simulink model "HW7_v1"  (R2019b)
settings: Solver=VariableStepAuto  StartTime=0.0  StopTime=15  RelTol=1e-3
values from neighbouring files (symbols this model uses):
  A1 = [0 1;        0 0]    [HW7_v1.m]
  A1_wiener = [0 1 ;               0 0]    [HW7_v1.m]
  A2 = [0 1 0 0;        0 0 0 0;        0 0 0 1;       -9.81 0 0 0]    [HW7_v1.m]
  A2_cont = [0]    [HW7_v1.m]
  A3 = [0 1 0 0;        0 0 0 0;        0 0 0 1;       9.81 0 0 0]    [HW7_v1.m]
  A4 = [0 1;        0 0]    [HW7_v1.m]
  B1 = [0;      -0.067]    [HW7_v1.m]
  B1_wiener = [0;               1]    [HW7_v1.m]
  B2 = [0;        0.1442 ... (first row only)    [HW7_v1.m]
  B2_cont = [1]    [HW7_v1.m]
  B3 = [0;        0.1774;        0;        0]    [HW7_v1.m]
  B4 = [0;       0.1728]    [HW7_v1.m]
  C1 = [1 0]    [HW7_v1.m]
  C1_wiener = [1 0]    [HW7_v1.m]
  C2 = [1 0 0 0;        0 1 0 0;        0 0 1 0;        0 0 0 1]    [HW7_v1.m]
  C2_cont = [1]    [HW7_v1.m]
  C3 = [1 0 0 0;        0 1 0 0;        0 0 1 0;        0 0 0 1]    [HW7_v1.m]
  C4 = [1 0;        0 1]    [HW7_v1.m]
  D1 = [0]    [HW7_v1.m]
  D1_wiener = [0]    [HW7_v1.m]
  D2 = [0;        0;        0;        0]    [HW7_v1.m]
  D2_cont = [0]    [HW7_v1.m]
  D3 = [0;        0;        0;        0]    [HW7_v1.m]
  D4 = [0;       0]    [HW7_v1.m]
  Kx1 = K1(2:3)    [HW7_v1.m]
  L1 = lqe(A1_cont, G1, C1_cont, Q1, R1, N1)    [HW7_v1.m]
  L2 = lqe(A2_cont, G2, C2_cont, Q2, R2, N2)    [HW7_v1.m]
  L3 = lqe(A2_cont, G2, C2_cont, Q3, R3, N3)    [HW7_v1.m]
  L4 = lqe(A2_cont, G2, C2_cont, Q4, R4, N4)    [HW7_v1.m]
  L5 = lqe(A2_cont, G2, C2_cont, Q5, R5, N5)    [HW7_v1.m]
  M_inv = inv(M_motor)    [HW7_v1.m]
  M_motor = [1, 1, 1, -1;             1, 1, -1, 1;             1, -1, -1, -1;             1, -1, 1, 1 ]    [HW7_v1.m]
  tau2 = eval(max(solve(1/sqrt((tau2*2*pi*10)^2+1^2) == 1/sqrt(2), tau2)))    [HW7_v1.m]
  V = 5    [HW7_v1.m]
  V0 = 5    [HW7_v1.m]
undefined symbols (not defined in the file or in its folder): DiscIntNeverNeededParam, K2, K3, K4
settings Model: Creator=cwhipp  LastModifiedBy=cwhipp

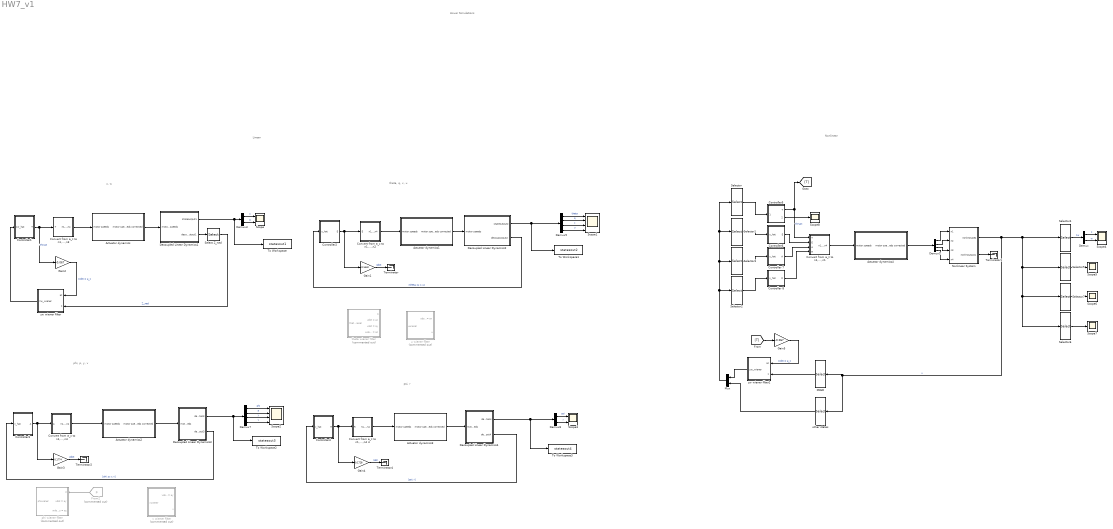
== system HW7_v1 ==
  note: Hover Simulations
  note: Nonlinear
  note: Linear
  note: z, w
  note: theta, q, x, u
  note: phi, p, y, v
  note: psi, r
  Actuator dynamics : Subsystem
  Actuator dynamics1 : Subsystem
  Actuator dynamics2 : Subsystem
  Actuator dynamics3 : Subsystem
  Actuator dynamics4 : Subsystem
  Controller 7 : Subsystem
  Controller 8 : Subsystem
  Controller1 : Subsystem
  Controller2 : Subsystem
  Controller3 : Subsystem
  Controller4 : Subsystem
  Controller5 : Subsystem
  Controller6 : Subsystem
  Convert from a_z to n1,...,n1 : Subsystem
  Convert from a_z to n1,...,n2 : Subsystem
  Convert from a_z to n1,...,n3 : Subsystem
  Convert from a_z to n1,...,n4 : Subsystem
  Convert from a_z to n1,...,n4 4 : Subsystem
  Decoupled Linear Dynamics1 : Subsystem
  Decoupled Linear Dynamics2 : Subsystem
  Decoupled Linear Dynamics3 : Subsystem
  "Decoupled Linear Dynamics4 " : Subsystem
  Demux : Demux  Outputs=2
  Demux1 : Demux
  Demux3 : Demux  Outputs=2
  Demux5 : Demux
  Demux7 : Demux
  Demux8 : Demux  Outputs=2
  From2 : From  Commented=on  GotoTag=p  TagVisibility=global
  Gain1 : Gain  Gain=0.1442
  Gain2 : Gain  Gain=-0.067
  Gain3 : Gain  Gain=0.1774
  Gain4 : Gain  Gain=0.1728
  Gain5 : Gain  Gain=-0.067
  Mux : Mux  Inputs=2
  Nonlinear System : Subsystem
  Scope : Scope  NumInputPorts=2
  Scope1 : Scope  NumInputPorts=4
  Scope2 : Scope  NumInputPorts=4
  Scope3 : Scope  NumInputPorts=2
  Scope4 : Scope  NumInputPorts=2
  Scope{5..8} (4 alike) : Scope
  Select Z_ned : Selector  InputPortWidth=4  IndexOptions=Index vector (dialog)  Indices=[1]  OutputSizes=1
  Selector : Selector  InputPortWidth=12  IndexOptions=Index vector (dialog)  Indices=[1 2]  OutputSizes=1
  Selector1 : Selector  InputPortWidth=12  IndexOptions=Index vector (dialog)  Indices=[3 4 5 6]  OutputSizes=1
  Selector2 : Selector  InputPortWidth=12  IndexOptions=Index vector (dialog)  Indices=[11 12]  OutputSizes=1
  Selector3 : Selector  InputPortWidth=12  IndexOptions=Index vector (dialog)  Indices=[7 8 9 10]  OutputSizes=1
  Selector4 : Selector  InputPortWidth=12  IndexOptions=Index vector (dialog)  Indices=[1 2]  OutputSizes=1
  Selector5 : Selector  InputPortWidth=12  IndexOptions=Index vector (dialog)  Indices=[3 4 5 6]  OutputSizes=1
  Selector6 : Selector  InputPortWidth=12  IndexOptions=Index vector (dialog)  Indices=[11 12]  OutputSizes=1
  Selector7 : Selector  InputPortWidth=12  IndexOptions=Index vector (dialog)  Indices=[7 8 9 10]  OutputSizes=1
  Terminator{,1..2,4} (4 alike) : Terminator
  To Workspace : ToWorkspace  VariableName=statesout1  SaveFormat=Timeseries  SampleTime=-1
  To Workspace1 : ToWorkspace  VariableName=statesout2  SaveFormat=Timeseries  SampleTime=-1
  To Workspace2 : ToWorkspace  VariableName=statesout3  SaveFormat=Timeseries  SampleTime=-1
  To Workspace3 : ToWorkspace  VariableName=statesout4  SaveFormat=Timeseries  SampleTime=-1
  ZNED : Selector  InputPortWidth=12  IndexOptions=Index vector (dialog)  Indices=[1]  OutputSizes=1
  other states : Selector  InputPortWidth=12  IndexOptions=Index vector (dialog)  Indices=[3 4 5 6 7 8 9 10 11 12]  OutputSizes=1
  phi wiener filter : Subsystem  Commented=on
  theta wiener filter : Subsystem  Commented=on
  u wiener filter : Subsystem  Commented=on
  v wiener filter : Subsystem  Commented=on
  zw wiener filter : Subsystem
  zw wiener filter2 : Subsystem
  wires:
  Gain5/1 -> zw wiener filter2/1(az)  "wdot = a_z"
  Demux1/1 -> Nonlinear System/1("n1 ")
  Demux1/2 -> Nonlinear System/2(n2)
  Demux1/3 -> Nonlinear System/3(n3)
  Demux1/4 -> Nonlinear System/4(n4)
  Controller1/1(T) -> Convert from a_z to n1,...,n3/1(T), Gain2/1  "thrust"
  Gain2/1 -> zw wiener filter/1(az)  "wdot = a_z"
  Select Z_ned/1 -> zw wiener filter/2(z)  "Z_ned"
  zw wiener filter/1(zw_wiener) -> Controller1/1(zw_hat)
  Decoupled Linear Dynamics1/2(decoupoutput1) -> Select Z_ned/1
  Decoupled Linear Dynamics2/2(decoupoutput2) -> Controller2/1(x_hat)  "[theta; q; x; u]"
  Controller2/1(E) -> Convert from a_z to n1,...,n2/1(E), Gain1/1
  Convert from a_z to n1,...,n2/1(n1,...,n4) -> Actuator dynamics1/1(motor speeds)
  Gain1/1 -> Terminator/1  "qdot"
  Decoupled Linear Dynamics3/2(decoupoutput3) -> Controller3/1(x_hat)  "[phi; p; y; v]"
  Gain3/1 -> Terminator2/1  "pdot"
  Convert from a_z to n1,...,n4/1(n1,...,n4) -> Actuator dynamics2/1(motor speeds)
  Controller3/1(A) -> Convert from a_z to n1,...,n4/1(A), Gain3/1
  From2/1 -> phi wiener filter/1(p)
  Controller4/1(R) -> Convert from a_z to n1,...,n4 4/1(R), Gain4/1
  Gain4/1 -> Terminator4/1  "rdot"
  Convert from a_z to n1,...,n4 4/1(n1,...,n4) -> Actuator dynamics3/1(motor speeds)
  "Decoupled Linear Dynamics4 "/2(decoupoutput4) -> Controller4/1(x_hat)  "[psi; r]"
  Decoupled Linear Dynamics1/1(stateoutput1) -> To Workspace/1, Demux3/1
  Demux3/1 -> Scope/1  "z"
  Demux3/2 -> Scope/2  "w"
  Demux5/4 -> Scope1/4  "u"
  Demux5/3 -> Scope1/3  "x"
  Demux5/2 -> Scope1/2  "q"
  Demux5/1 -> Scope1/1  "theta"
  Decoupled Linear Dynamics2/1(stateoutput2) -> To Workspace1/1, Demux5/1
  Demux7/2 -> Scope2/2  "p"
  Demux7/4 -> Scope2/4  "v"
  Demux7/1 -> Scope2/1  "phi"
  Demux7/3 -> Scope2/3  "y"
  Decoupled Linear Dynamics3/1(decoupstates3) -> To Workspace2/1, Demux7/1
  Demux8/2 -> Scope3/2  "r"
  Demux8/1 -> Scope3/1  "psi"
  "Decoupled Linear Dynamics4 "/1(decoupstates4) -> To Workspace3/1, Demux8/1
  Convert from a_z to n1,...,n3/1(n1,...,n4) -> Actuator dynamics/1(motor speeds)
  Actuator dynamics/1(motor speeds corrected) -> Decoupled Linear Dynamics1/1(motor speeds)
  Actuator dynamics1/1(motor speeds corrected) -> Decoupled Linear Dynamics2/1(motor speeds)
  Actuator dynamics2/1(motor speeds corrected) -> Decoupled Linear Dynamics3/1(motor speeds)
  Actuator dynamics3/1(motor speeds corrected) -> "Decoupled Linear Dynamics4 "/1(motor speeds)
  [T] -> Gain5/1
  Controller6/1(E) -> Convert from a_z to n1,...,n1/2(E)
  Controller 7/1(A) -> Convert from a_z to n1,...,n1/3(A)
  Controller 8/1(R) -> Convert from a_z to n1,...,n1/4(R)
  Selector1/1 -> Controller6/1(x_hat)
  Selector3/1 -> Controller 7/1(x_hat)
  Selector2/1 -> Controller 8/1(x_hat)
  Nonlinear System/2(nonlinoutputs) -> Terminator1/1
  ZNED/1 -> zw wiener filter2/2(z)
  zw wiener filter2/1(zw_wiener) -> Mux/1
  other states/1 -> Mux/2
  Mux/1 -> Selector/1, Selector1/1, Selector3/1, Selector2/1
  Nonlinear System/1("nonlinstates ") -> other states/1, ZNED/1, Selector6/1, Selector7/1, Selector5/1, Selector4/1  "x"
  Convert from a_z to n1,...,n1/1(n1,...,n4) -> Actuator dynamics4/1(motor speeds)
  Actuator dynamics4/1(motor speeds corrected) -> Demux1/1
  Selector4/1 -> Demux/1  "zw"
  Selector5/1 -> Scope5/1
  Selector7/1 -> Scope6/1
  Selector6/1 -> Scope7/1
  Controller5/1(T) -> Convert from a_z to n1,...,n1/1(T), [T]  "thrust"
  Selector/1 -> Controller5/1(zw_hat)
  Controller5/2(desired states) -> Scope8/1
  Demux/1 -> Scope4/1  "z"
  Demux/2 -> Scope4/2  "w"

== system HW7_v1/Actuator dynamics ==
  motor speeds : Inport
  30ms delay : TransportDelay  DelayTime=30e-3
  Demux : Demux
  Mux : Mux
  Saturation4 : Saturate  UpperLimit=500  LowerLimit=10
  Sum2 : Sum  Inputs=++|
  Transfer Fcn : TransferFcn  Denominator=[tau2 1]
  Transfer Fcn1 : TransferFcn  Denominator=[tau2 1]
  Transfer Fcn2 : TransferFcn  Denominator=[tau2 1]
  actuator transfer function : TransferFcn  Denominator=[tau2 1]
  speed correction : Constant  Value=299
  voltage correction : Gain  Gain=V/V0
  voltage error : Gain  Gain=V/V0
  motor speeds corrected : Outport
  wires:
  speed correction/1 -> Sum2/1
  voltage correction/1 -> voltage error/1
  Sum2/1 -> Saturation4/1
  Demux/2 -> Transfer Fcn1/1
  30ms delay/1 -> Demux/1
  Demux/4 -> actuator transfer function/1
  Demux/1 -> Transfer Fcn/1
  Demux/3 -> Transfer Fcn2/1
  voltage error/1 -> 30ms delay/1
  motor speeds/1 -> voltage correction/1
  Saturation4/1 -> motor speeds corrected/1
  Transfer Fcn/1 -> Mux/1
  Transfer Fcn1/1 -> Mux/2
  Transfer Fcn2/1 -> Mux/3
  actuator transfer function/1 -> Mux/4
  Mux/1 -> Sum2/2

== system HW7_v1/Actuator dynamics1 ==
  motor speeds : Inport
  30ms delay : TransportDelay  DelayTime=30e-3
  Demux : Demux
  Mux : Mux
  Saturation4 : Saturate  UpperLimit=500  LowerLimit=10
  Sum2 : Sum  Inputs=++|
  Transfer Fcn : TransferFcn  Denominator=[tau2 1]
  Transfer Fcn1 : TransferFcn  Denominator=[tau2 1]
  Transfer Fcn2 : TransferFcn  Denominator=[tau2 1]
  actuator transfer function : TransferFcn  Denominator=[tau2 1]
  speed correction : Constant  Value=299
  voltage correction : Gain  Gain=V/V0
  voltage error : Gain  Gain=V/V0
  motor speeds corrected : Outport
  wires:
  speed correction/1 -> Sum2/1
  voltage correction/1 -> voltage error/1
  Sum2/1 -> Saturation4/1
  Demux/2 -> Transfer Fcn1/1
  30ms delay/1 -> Demux/1
  Demux/4 -> actuator transfer function/1
  Demux/1 -> Transfer Fcn/1
  Demux/3 -> Transfer Fcn2/1
  voltage error/1 -> 30ms delay/1
  motor speeds/1 -> voltage correction/1
  Saturation4/1 -> motor speeds corrected/1
  Transfer Fcn/1 -> Mux/1
  Transfer Fcn1/1 -> Mux/2
  Transfer Fcn2/1 -> Mux/3
  actuator transfer function/1 -> Mux/4
  Mux/1 -> Sum2/2

== system HW7_v1/Actuator dynamics2 ==
  motor speeds : Inport
  30ms delay : TransportDelay  DelayTime=30e-3
  Demux : Demux
  Mux : Mux
  Saturation4 : Saturate  UpperLimit=500  LowerLimit=10
  Sum2 : Sum  Inputs=++|
  Transfer Fcn : TransferFcn  Denominator=[tau2 1]
  Transfer Fcn1 : TransferFcn  Denominator=[tau2 1]
  Transfer Fcn2 : TransferFcn  Denominator=[tau2 1]
  actuator transfer function : TransferFcn  Denominator=[tau2 1]
  speed correction : Constant  Value=299
  voltage correction : Gain  Gain=V/V0
  voltage error : Gain  Gain=V/V0
  motor speeds corrected : Outport
  wires:
  speed correction/1 -> Sum2/1
  voltage correction/1 -> voltage error/1
  Sum2/1 -> Saturation4/1
  Demux/2 -> Transfer Fcn1/1
  30ms delay/1 -> Demux/1
  Demux/4 -> actuator transfer function/1
  Demux/1 -> Transfer Fcn/1
  Demux/3 -> Transfer Fcn2/1
  voltage error/1 -> 30ms delay/1
  motor speeds/1 -> voltage correction/1
  Saturation4/1 -> motor speeds corrected/1
  Transfer Fcn/1 -> Mux/1
  Transfer Fcn1/1 -> Mux/2
  Transfer Fcn2/1 -> Mux/3
  actuator transfer function/1 -> Mux/4
  Mux/1 -> Sum2/2

== system HW7_v1/Actuator dynamics3 ==
  motor speeds : Inport
  30ms delay : TransportDelay  DelayTime=30e-3
  Demux : Demux
  Mux : Mux
  Saturation4 : Saturate  UpperLimit=500  LowerLimit=10
  Sum2 : Sum  Inputs=++|
  Transfer Fcn : TransferFcn  Denominator=[tau2 1]
  Transfer Fcn1 : TransferFcn  Denominator=[tau2 1]
  Transfer Fcn2 : TransferFcn  Denominator=[tau2 1]
  actuator transfer function : TransferFcn  Denominator=[tau2 1]
  speed correction : Constant  Value=299
  voltage correction : Gain  Gain=V/V0
  voltage error : Gain  Gain=V/V0
  motor speeds corrected : Outport
  wires:
  speed correction/1 -> Sum2/1
  voltage correction/1 -> voltage error/1
  Sum2/1 -> Saturation4/1
  Demux/2 -> Transfer Fcn1/1
  30ms delay/1 -> Demux/1
  Demux/4 -> actuator transfer function/1
  Demux/1 -> Transfer Fcn/1
  Demux/3 -> Transfer Fcn2/1
  voltage error/1 -> 30ms delay/1
  motor speeds/1 -> voltage correction/1
  Saturation4/1 -> motor speeds corrected/1
  Transfer Fcn/1 -> Mux/1
  Transfer Fcn1/1 -> Mux/2
  Transfer Fcn2/1 -> Mux/3
  actuator transfer function/1 -> Mux/4
  Mux/1 -> Sum2/2

== system HW7_v1/Actuator dynamics4 ==
  motor speeds : Inport
  30ms delay : TransportDelay  DelayTime=30e-3
  Demux : Demux
  Mux : Mux
  Saturation4 : Saturate  UpperLimit=500  LowerLimit=10
  Sum2 : Sum  Inputs=++|
  Transfer Fcn : TransferFcn  Denominator=[tau2 1]
  Transfer Fcn1 : TransferFcn  Denominator=[tau2 1]
  Transfer Fcn2 : TransferFcn  Denominator=[tau2 1]
  actuator transfer function : TransferFcn  Denominator=[tau2 1]
  speed correction : Constant  Value=299
  voltage correction : Gain  Gain=V/V0
  voltage error : Gain  Gain=V/V0
  motor speeds corrected : Outport
  wires:
  speed correction/1 -> Sum2/1
  voltage correction/1 -> voltage error/1
  Sum2/1 -> Saturation4/1
  Demux/2 -> Transfer Fcn1/1
  30ms delay/1 -> Demux/1
  Demux/4 -> actuator transfer function/1
  Demux/1 -> Transfer Fcn/1
  Demux/3 -> Transfer Fcn2/1
  voltage error/1 -> 30ms delay/1
  motor speeds/1 -> voltage correction/1
  Saturation4/1 -> motor speeds corrected/1
  Transfer Fcn/1 -> Mux/1
  Transfer Fcn1/1 -> Mux/2
  Transfer Fcn2/1 -> Mux/3
  actuator transfer function/1 -> Mux/4
  Mux/1 -> Sum2/2

== system HW7_v1/Controller 7 ==
  x_hat : Inport
  Sum : Sum  Inputs=+-|
  controller gain : Gain  Gain=K3  Multiplication=Matrix(K*u)
  desired velocity : Constant  Value=[0; 0; 0; 0]  SampleTime=0.05
  A : Outport
  wires:
  controller gain/1 -> A/1  "u = K(x-x)"
  x_hat/1 -> Sum/2
  Sum/1 -> controller gain/1
  desired velocity/1 -> Sum/1

== system HW7_v1/Controller 8 ==
  x_hat : Inport
  Sum : Sum  Inputs=+-|
  controller gain : Gain  Gain=K4  Multiplication=Matrix(K*u)
  desired velocity : Constant  Value=[0; 0]  SampleTime=0.05
  R : Outport
  wires:
  controller gain/1 -> R/1  "u = K(x-x)"
  x_hat/1 -> Sum/2
  Sum/1 -> controller gain/1
  desired velocity/1 -> Sum/1

== system HW7_v1/Controller1 ==
  zw_hat : Inport
  Constant1 : Constant  Value=1.5  SampleTime=0.05
  Gain : Gain  Gain=Kx1  Multiplication=Matrix(K*u)
  Gain1 : Gain  Gain=-1
  Mux : Mux  Inputs=2
  Scope : Scope
  Sum : Sum  Inputs=+-|
  Sum1 : Sum  Inputs=++|
  desired position : DiscretePulseGenerator  PulseType=Time based  Amplitude=-1.5  Period=10  PulseWidth=50
  desired velocity : Constant  Value=0  SampleTime=0.05
  T : Outport
  wires:
  Gain/1 -> T/1  "u = K(x-x)"
  zw_hat/1 -> Sum/2
  Sum/1 -> Gain/1
  Constant1/1 -> Sum1/1
  desired position/1 -> Sum1/2
  Sum1/1 -> Gain1/1
  Gain1/1 -> Mux/1
  desired velocity/1 -> Mux/2
  Mux/1 -> Scope/1, Sum/1

== system HW7_v1/Controller2 ==
  x_hat : Inport
  Sum : Sum  Inputs=+-|
  controller gain : Gain  Gain=K2  Multiplication=Matrix(K*u)
  desired velocity : Constant  Value=[0; 0; 0; 0]  SampleTime=0.05
  E : Outport
  wires:
  controller gain/1 -> E/1  "u = K(x-x)"
  x_hat/1 -> Sum/2
  Sum/1 -> controller gain/1
  desired velocity/1 -> Sum/1

== system HW7_v1/Controller3 ==
  x_hat : Inport
  Sum : Sum  Inputs=+-|
  controller gain : Gain  Gain=K3  Multiplication=Matrix(K*u)
  desired velocity : Constant  Value=[0; 0; 0; 0]  SampleTime=0.05
  A : Outport
  wires:
  controller gain/1 -> A/1  "u = K(x-x)"
  x_hat/1 -> Sum/2
  Sum/1 -> controller gain/1
  desired velocity/1 -> Sum/1

== system HW7_v1/Controller4 ==
  x_hat : Inport
  Sum : Sum  Inputs=+-|
  controller gain : Gain  Gain=K4  Multiplication=Matrix(K*u)
  desired velocity : Constant  Value=[0; 0]  SampleTime=0.05
  R : Outport
  wires:
  controller gain/1 -> R/1  "u = K(x-x)"
  x_hat/1 -> Sum/2
  Sum/1 -> controller gain/1
  desired velocity/1 -> Sum/1

== system HW7_v1/Controller5 ==
  zw_hat : Inport
  Constant1 : Constant  Value=1.5  SampleTime=0.05
  Gain : Gain  Gain=Kx1  Multiplication=Matrix(K*u)
  Gain1 : Gain  Gain=-1
  Mux : Mux  Inputs=2
  Sum : Sum  Inputs=+-|
  Sum1 : Sum  Inputs=++|
  desired position : DiscretePulseGenerator  PulseType=Time based  Amplitude=-1.5  Period=10  PulseWidth=50
  desired velocity : Constant  Value=0  SampleTime=0.05
  T : Outport
  desired states : Outport  Port=2
  wires:
  Gain/1 -> T/1  "u = K(x-x)"
  zw_hat/1 -> Sum/2
  Sum/1 -> Gain/1
  Constant1/1 -> Sum1/1
  desired position/1 -> Sum1/2
  Sum1/1 -> Gain1/1
  Gain1/1 -> Mux/1
  desired velocity/1 -> Mux/2
  Mux/1 -> Sum/1, desired states/1

== system HW7_v1/Controller6 ==
  x_hat : Inport
  Sum : Sum  Inputs=+-|
  controller gain : Gain  Gain=K2  Multiplication=Matrix(K*u)
  desired velocity : Constant  Value=[0; 0; 0; 0]  SampleTime=0.05
  E : Outport
  wires:
  controller gain/1 -> E/1  "u = K(x-x)"
  x_hat/1 -> Sum/2
  Sum/1 -> controller gain/1
  desired velocity/1 -> Sum/1

== system HW7_v1/Convert from a_z to n1,...,n1 ==
  T : Inport
  E : Inport  Port=2
  A : Inport  Port=3
  R : Inport  Port=4
  Convert fom TEAR to n1,..,n4 : Gain  Gain=M_motor  Multiplication=Matrix(K*u)
  Mux : Mux
  n1,...,n4 : Outport
  wires:
  Convert fom TEAR to n1,..,n4/1 -> n1,...,n4/1
  Mux/1 -> Convert fom TEAR to n1,..,n4/1
  T/1 -> Mux/1
  E/1 -> Mux/2
  A/1 -> Mux/3
  R/1 -> Mux/4

== system HW7_v1/Convert from a_z to n1,...,n2 ==
  E : Inport
  Constant : Constant  Value=0
  Convert fom TEAR to n1,..,n4 : Gain  Gain=M_motor  Multiplication=Matrix(K*u)
  Mux : Mux
  n1,...,n4 : Outport
  wires:
  Constant/1 -> Mux/4, Mux/1, Mux/3
  Convert fom TEAR to n1,..,n4/1 -> n1,...,n4/1
  Mux/1 -> Convert fom TEAR to n1,..,n4/1
  E/1 -> Mux/2

== system HW7_v1/Convert from a_z to n1,...,n3 ==
  T : Inport
  Constant : Constant  Value=0
  Convert fom TEAR to n1,..,n4 : Gain  Gain=M_motor  Multiplication=Matrix(K*u)
  Mux : Mux
  n1,...,n4 : Outport
  wires:
  Constant/1 -> Mux/4, Mux/3, Mux/2
  Convert fom TEAR to n1,..,n4/1 -> n1,...,n4/1
  Mux/1 -> Convert fom TEAR to n1,..,n4/1
  T/1 -> Mux/1

== system HW7_v1/Convert from a_z to n1,...,n4 ==
  A : Inport
  Constant : Constant  Value=0
  Convert fom TEAR to n1,..,n4 : Gain  Gain=M_motor  Multiplication=Matrix(K*u)
  Mux : Mux
  n1,...,n4 : Outport
  wires:
  Constant/1 -> Mux/4, Mux/2, Mux/1
  Convert fom TEAR to n1,..,n4/1 -> n1,...,n4/1
  Mux/1 -> Convert fom TEAR to n1,..,n4/1
  A/1 -> Mux/3

== system HW7_v1/Convert from a_z to n1,...,n4 4 ==
  R : Inport
  Constant : Constant  Value=0
  Convert fom TEAR to n1,..,n4 : Gain  Gain=M_motor  Multiplication=Matrix(K*u)
  Mux : Mux
  n1,...,n4 : Outport
  wires:
  Constant/1 -> Mux/3, Mux/2, Mux/1
  Convert fom TEAR to n1,..,n4/1 -> n1,...,n4/1
  Mux/1 -> Convert fom TEAR to n1,..,n4/1
  R/1 -> Mux/4

== system HW7_v1/Decoupled Linear Dynamics1 ==
  motor speeds : Inport
  B*u : Gain  Gain=B1  Multiplication=Matrix(K*u)
  Demux : Demux
  Gain : Gain  Gain=M_inv  Multiplication=Matrix(K*u)
  Gain2 : Gain  Gain=C1  Multiplication=Matrix(K*u)
  Gain3 : Gain  Gain=D1  Multiplication=Matrix(K*u)
  Gain69 : Gain  Gain=A1  Multiplication=Matrix(K*u)
  Integrator : Integrator
  Selector : Selector  InputPortWidth=4  IndexOptions=Index vector (dialog)  Indices=1  OutputSizes=1
  Sum : Sum  Inputs=|++
  Sum1 : Sum  Inputs=|++
  Sum4 : Sum  Inputs=-+|
  asdf : Scope  NumInputPorts=4
  change back to trim = 0 : Constant  Value=299
  stateoutput1 : Outport
  decoupoutput1 : Outport  Port=2
  wires:
  Sum/1 -> Integrator/1
  Gain69/1 -> Sum/2  "Ax"
  Gain3/1 -> Sum1/1  "Du"
  Sum1/1 -> decoupoutput1/1  "y"
  B*u/1 -> Sum/1
  Gain2/1 -> Sum1/2  "Cx"
  Selector/1 -> Gain3/1, B*u/1  "u"
  Gain/1 -> Selector/1
  Integrator/1 -> Gain2/1, stateoutput1/1, Gain69/1  "x"
  change back to trim = 0/1 -> Sum4/1
  Demux/1 -> asdf/1
  Demux/2 -> asdf/2
  Demux/3 -> asdf/3
  Sum4/1 -> Demux/1, Gain/1
  motor speeds/1 -> Sum4/2
  Demux/4 -> asdf/4

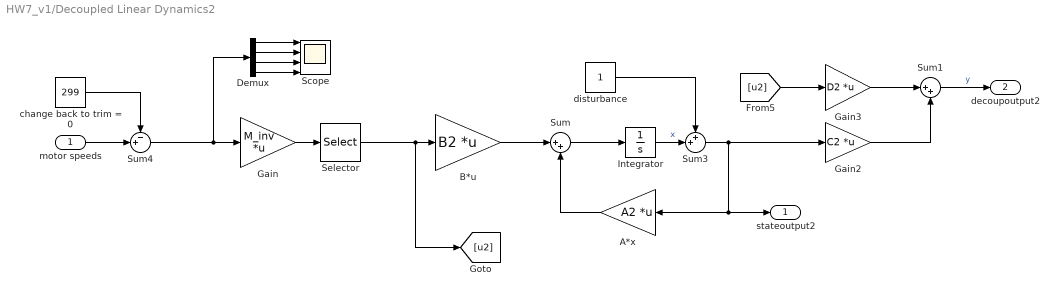
== system HW7_v1/Decoupled Linear Dynamics2 ==
  motor speeds : Inport
  A*x : Gain  Gain=A2  Multiplication=Matrix(K*u)
  B*u : Gain  Gain=B2  Multiplication=Matrix(K*u)
  Demux : Demux
  Gain : Gain  Gain=M_inv  Multiplication=Matrix(K*u)
  Gain2 : Gain  Gain=C2  Multiplication=Matrix(K*u)
  Gain3 : Gain  Gain=D2  Multiplication=Matrix(K*u)
  Integrator : Integrator
  Scope : Scope  NumInputPorts=4
  Selector : Selector  InputPortWidth=4  IndexOptions=Index vector (dialog)  Indices=2  OutputSizes=1
  Sum : Sum  Inputs=|++
  Sum1 : Sum  Inputs=|++
  Sum3 : Sum  Inputs=++|
  Sum4 : Sum  Inputs=-+|
  change back to trim = 0 : Constant  Value=299
  disturbance : Constant
  stateoutput2 : Outport
  decoupoutput2 : Outport  Port=2
  wires:
  Sum/1 -> Integrator/1
  A*x/1 -> Sum/2
  Gain3/1 -> Sum1/1
  Sum1/1 -> decoupoutput2/1  "y"
  B*u/1 -> Sum/1
  Gain2/1 -> Sum1/2
  [u2] -> Gain3/1
  Sum4/1 -> Demux/1, Gain/1
  Gain/1 -> Selector/1
  Selector/1 -> [u2], B*u/1
  change back to trim = 0/1 -> Sum4/1
  Demux/1 -> Scope/1
  Demux/2 -> Scope/2
  Demux/3 -> Scope/3
  Demux/4 -> Scope/4
  motor speeds/1 -> Sum4/2
  disturbance/1 -> Sum3/1
  Integrator/1 -> Sum3/2  "x"
  Sum3/1 -> stateoutput2/1, A*x/1, Gain2/1

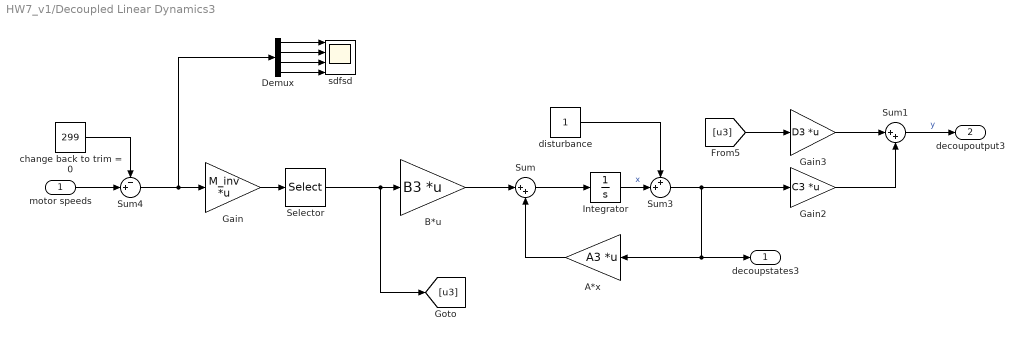
== system HW7_v1/Decoupled Linear Dynamics3 ==
  motor speeds : Inport
  A*x : Gain  Gain=A3  Multiplication=Matrix(K*u)
  B*u : Gain  Gain=B3  Multiplication=Matrix(K*u)
  Demux : Demux
  Gain : Gain  Gain=M_inv  Multiplication=Matrix(K*u)
  Gain2 : Gain  Gain=C3  Multiplication=Matrix(K*u)
  Gain3 : Gain  Gain=D3  Multiplication=Matrix(K*u)
  Integrator : Integrator
  Selector : Selector  InputPortWidth=4  IndexOptions=Index vector (dialog)  Indices=3  OutputSizes=1
  Sum : Sum  Inputs=|++
  Sum1 : Sum  Inputs=|++
  Sum3 : Sum  Inputs=++|
  Sum4 : Sum  Inputs=-+|
  change back to trim = 0 : Constant  Value=299
  disturbance : Constant
  sdfsd : Scope  NumInputPorts=4
  decoupstates3 : Outport
  decoupoutput3 : Outport  Port=2
  wires:
  Sum/1 -> Integrator/1
  A*x/1 -> Sum/2
  Gain3/1 -> Sum1/1
  Sum1/1 -> decoupoutput3/1  "y"
  B*u/1 -> Sum/1
  Gain2/1 -> Sum1/2
  [u3] -> Gain3/1
  Sum4/1 -> Demux/1, Gain/1
  Gain/1 -> Selector/1
  Selector/1 -> [u3], B*u/1
  change back to trim = 0/1 -> Sum4/1
  Demux/1 -> sdfsd/1
  Demux/2 -> sdfsd/2
  Demux/3 -> sdfsd/3
  Demux/4 -> sdfsd/4
  motor speeds/1 -> Sum4/2
  disturbance/1 -> Sum3/1
  Integrator/1 -> Sum3/2  "x"
  Sum3/1 -> decoupstates3/1, A*x/1, Gain2/1

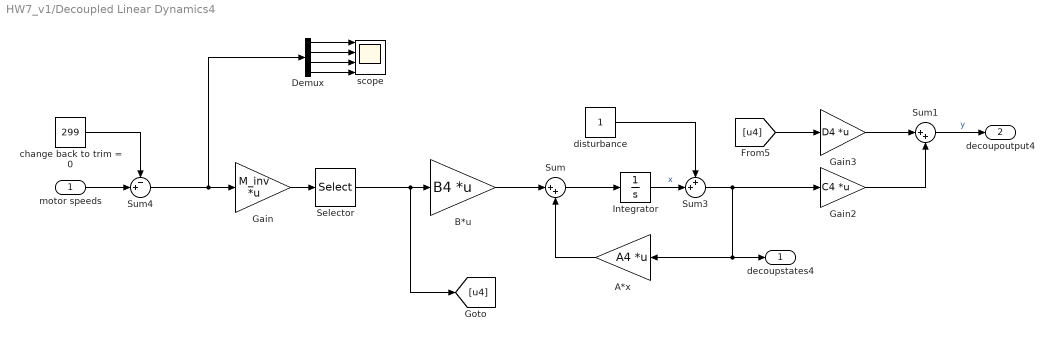
== system HW7_v1/Decoupled Linear Dynamics4  ==
  motor speeds : Inport
  A*x : Gain  Gain=A4  Multiplication=Matrix(K*u)
  B*u : Gain  Gain=B4  Multiplication=Matrix(K*u)
  Demux : Demux
  Gain : Gain  Gain=M_inv  Multiplication=Matrix(K*u)
  Gain2 : Gain  Gain=C4  Multiplication=Matrix(K*u)
  Gain3 : Gain  Gain=D4  Multiplication=Matrix(K*u)
  Integrator : Integrator
  Selector : Selector  InputPortWidth=4  IndexOptions=Index vector (dialog)  Indices=4  OutputSizes=1
  Sum : Sum  Inputs=|++
  Sum1 : Sum  Inputs=|++
  Sum3 : Sum  Inputs=++|
  Sum4 : Sum  Inputs=-+|
  change back to trim = 0 : Constant  Value=299
  disturbance : Constant
  scope : Scope  NumInputPorts=4
  decoupstates4 : Outport
  decoupoutput4 : Outport  Port=2
  wires:
  Sum/1 -> Integrator/1
  A*x/1 -> Sum/2
  Gain3/1 -> Sum1/1
  Sum1/1 -> decoupoutput4/1  "y"
  B*u/1 -> Sum/1
  Gain2/1 -> Sum1/2
  [u4] -> Gain3/1
  Sum4/1 -> Demux/1, Gain/1
  Gain/1 -> Selector/1
  Selector/1 -> [u4], B*u/1
  change back to trim = 0/1 -> Sum4/1
  Demux/1 -> scope/1
  Demux/2 -> scope/2
  Demux/3 -> scope/3
  Demux/4 -> scope/4
  Sum3/1 -> decoupstates4/1, A*x/1, Gain2/1
  motor speeds/1 -> Sum4/2
  disturbance/1 -> Sum3/1
  Integrator/1 -> Sum3/2  "x"

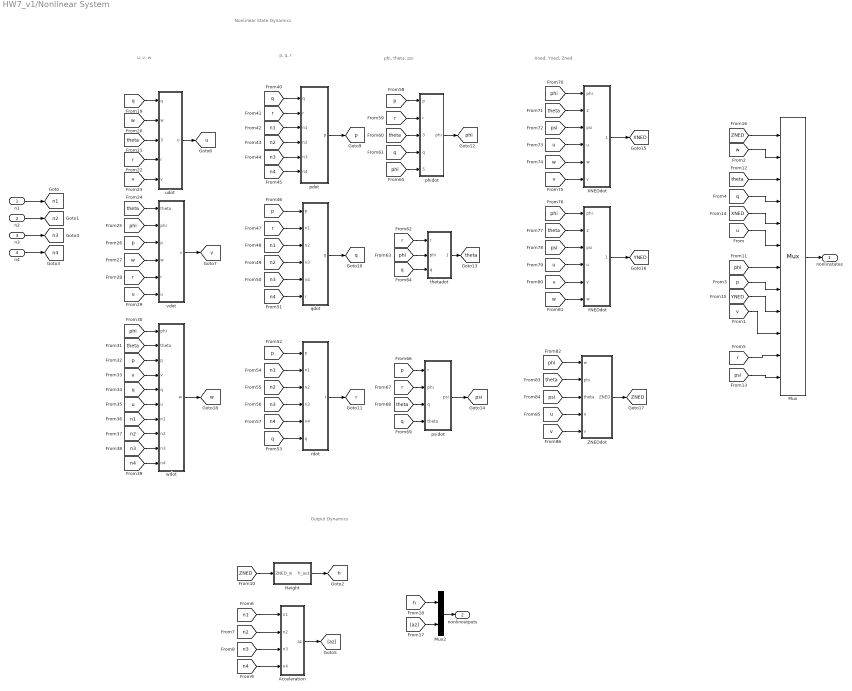
== system HW7_v1/Nonlinear System ==
  note: Output Dynamics
  note: Nonlinear State Dynamics
  note: p, q, r
  note: u, v, w
  note: phi, theta, psi
  note: Xned, Yned, Zned
  "n1 " : Inport
  n2 : Inport  Port=2
  n3 : Inport  Port=3
  n4 : Inport  Port=4
  Acceleration : Subsystem
  Height : Subsystem
  Mux : Mux  Inputs=12
  Mux2 : Mux  Inputs=2
  "XNEDdot " : Subsystem
  "YNEDdot " : Subsystem
  ZNEDdot : Subsystem
  pdot : Subsystem
  phidot : Subsystem
  "psidot " : Subsystem
  qdot : Subsystem
  rdot : Subsystem
  "thetadot " : Subsystem
  udot : Subsystem
  vdot : Subsystem
  "wdot " : Subsystem
  "nonlinstates " : Outport
  nonlinoutputs : Outport  Port=2
  tag scope: XNED=global, YNED=global, ZNED=global, h=global, n1=global, n2=global, n3=global, n4=global, p=global, phi=global, psi=global, q=global, r=global, theta=global, u=global, v=global, w=global
  wires:
  [n2] -> Acceleration/2(n2)
  [n1] -> Acceleration/1(n1)
  [n3] -> Acceleration/3(n3)
  Acceleration/1(az) -> [az]
  [n4] -> Acceleration/4(n4)
  [ZNED] -> Height/1("ZNED_in ")
  Height/1("h_out ") -> [h]
  Mux/1 -> "nonlinstates "/1
  [h] -> Mux2/1
  [az] -> Mux2/2
  Mux2/1 -> nonlinoutputs/1
  udot/1("u ") -> [u]
  [q] -> udot/1("q ")
  [w] -> udot/2("w ")
  [theta] -> udot/3(theta)
  [r] -> udot/4("r ")
  [v] -> udot/5(v)
  "n1 "/1 -> [n1]
  n2/1 -> [n2]
  n3/1 -> [n3]
  n4/1 -> [n4]
  [theta] -> vdot/1(theta)
  [phi] -> vdot/2(phi)
  [p] -> vdot/3(p)
  [w] -> vdot/4(w)
  [r] -> vdot/5(r)
  [u] -> vdot/6(u)
  vdot/1(v) -> [v]
  [phi] -> "wdot "/1(phi)
  [theta] -> "wdot "/2(theta)
  [p] -> "wdot "/3(p)
  [v] -> "wdot "/4(v)
  [q] -> "wdot "/5(q)
  [u] -> "wdot "/6(u)
  [n1] -> "wdot "/7(n1)
  [n2] -> "wdot "/8(n2)
  [n3] -> "wdot "/9(n3)
  [n4] -> "wdot "/10(n4)
  "wdot "/1(w) -> [w]
  [n1] -> pdot/3(n1)
  [r] -> pdot/2(r)
  [n2] -> pdot/4(n2)
  [q] -> pdot/1(q)
  [n3] -> pdot/5(n3)
  [n4] -> pdot/6(n4)
  [p] -> qdot/1(p)
  [r] -> qdot/2(n1)
  [n1] -> qdot/3(n2)
  [n2] -> qdot/4(n3)
  [n3] -> qdot/5(n4)
  [n4] -> qdot/6(r)
  qdot/1(q) -> [q]
  [p] -> rdot/1(p)
  [n1] -> rdot/2(n1)
  [n2] -> rdot/3(n2)
  [n3] -> rdot/4(n3)
  [n4] -> rdot/5(n4)
  [q] -> rdot/6(q)
  rdot/1(r) -> [r]
  [p] -> phidot/1(p)
  [r] -> phidot/2(r)
  [theta] -> phidot/3(theta)
  [q] -> phidot/4(q)
  phidot/1(phi) -> [phi]
  [q] -> "thetadot "/3(q)
  [r] -> "thetadot "/1(r)
  [phi] -> "thetadot "/2(phi)
  "thetadot "/1(theta) -> [theta]
  pdot/1(p) -> [p]
  [phi] -> phidot/5(phi in)
  [r] -> "psidot "/2(phi)
  [p] -> "psidot "/1(r)
  [theta] -> "psidot "/3(q)
  [q] -> "psidot "/4(theta)
  "psidot "/1(psi) -> [psi]
  [phi] -> "XNEDdot "/1(phi)
  [u] -> "XNEDdot "/4(u)
  [w] -> "XNEDdot "/5(w)
  [v] -> "XNEDdot "/6(v)
  [theta] -> "XNEDdot "/2(theta)
  [psi] -> "XNEDdot "/3(psi)
  "XNEDdot "/1(XNED) -> [XNED]
  [w] -> "YNEDdot "/6(w)
  [v] -> "YNEDdot "/5(v)
  [u] -> "YNEDdot "/4(u)
  [psi] -> "YNEDdot "/3(psi)
  [theta] -> "YNEDdot "/2(theta)
  "YNEDdot "/1(YNED) -> [YNED]
  [phi] -> "YNEDdot "/1(phi)
  [phi] -> ZNEDdot/1(w)
  [theta] -> ZNEDdot/2(phi)
  [psi] -> ZNEDdot/3(theta)
  [u] -> ZNEDdot/4(u)
  [v] -> ZNEDdot/5(v)
  ZNEDdot/1(ZNED) -> [ZNED]
  [r] -> Mux/11
  [psi] -> Mux/12
  [phi] -> Mux/7
  [p] -> Mux/8
  [YNED] -> Mux/9
  [v] -> Mux/10
  [u] -> Mux/6
  [XNED] -> Mux/5
  [q] -> Mux/4
  [theta] -> Mux/3
  [w] -> Mux/2
  [ZNED] -> Mux/1

== system HW7_v1/phi wiener filter ==
  p : Inport
  vdot = ay : Inport  Port=2
  wdotnobias = az : Inport  Port=3
  Discrete-Time Integrator3 : DiscreteIntegrator  IntegratorMethod=Integration: Backward Euler  SampleTime=-1  ICPrevOutput=DiscIntNeverNeededParam  ICPrevScaledInput=DiscIntNeverNeededParam
  Divide2 : Product  Inputs=*/
  Gain16 : Gain  Gain=D2_cont  Multiplication=Matrix(K*u)
  Gain17 : Gain  Gain=A2_cont  Multiplication=Matrix(K*u)
  Gain18 : Gain  Gain=B2_cont  Multiplication=Matrix(K*u)
  Gain19 : Gain  Gain=L4  Multiplication=Matrix(K*u)
  Gain20 : Gain  Gain=C2_cont  Multiplication=Matrix(K*u)
  Memory4 : Memory
  Sum15 : Sum  Inputs=|+-
  Sum16 : Sum  Inputs=|++
  Sum17 : Sum  Inputs=|++
  Sum18 : Sum  Inputs=|+-
  phiwiener : Outport
  wires:
  Gain18/1 -> Sum16/2  "Bu"
  Gain17/1 -> Sum16/1  "Axe"
  Gain19/1 -> Sum17/2  "L(y-Cx-Du)"
  Sum18/1 -> Gain19/1
  Discrete-Time Integrator3/1 -> Gain17/1, phiwiener/1, Gain20/1  "xe"
  wdotnobias = az/1 -> Divide2/2
  Memory4/1 -> Discrete-Time Integrator3/1
  vdot = ay/1 -> Divide2/1
  Divide2/1 -> Sum15/1  "phi"
  p/1 -> Gain16/1, Gain18/1  "u"
  Sum15/1 -> Sum18/1
  Sum16/1 -> Sum17/1
  Sum17/1 -> Memory4/1
  Gain16/1 -> Sum15/2  "Du"
  Gain20/1 -> Sum18/2  "Cx"

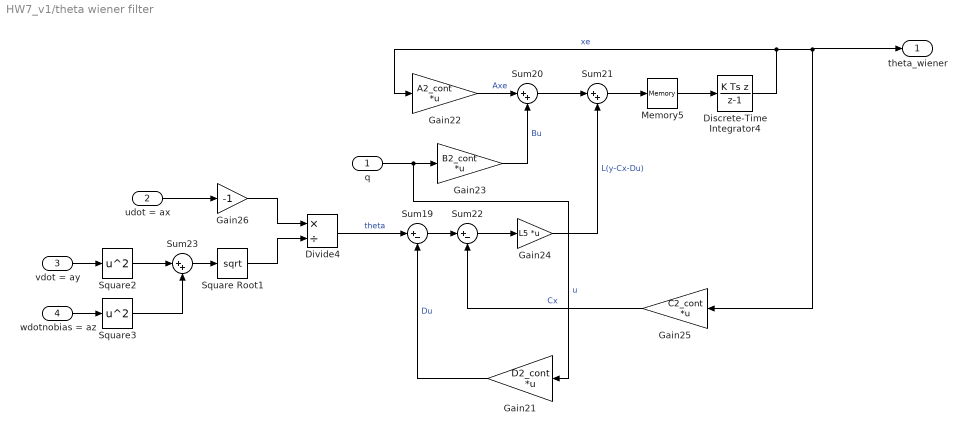
== system HW7_v1/theta wiener filter ==
  q : Inport
  udot = ax : Inport  Port=2
  vdot = ay : Inport  Port=3
  "wdotnobias = az " : Inport  Port=4
  Discrete-Time Integrator4 : DiscreteIntegrator  IntegratorMethod=Integration: Backward Euler  SampleTime=-1  ICPrevOutput=DiscIntNeverNeededParam  ICPrevScaledInput=DiscIntNeverNeededParam
  Divide4 : Product  Inputs=*/
  Gain21 : Gain  Gain=D2_cont  Multiplication=Matrix(K*u)
  Gain22 : Gain  Gain=A2_cont  Multiplication=Matrix(K*u)
  Gain23 : Gain  Gain=B2_cont  Multiplication=Matrix(K*u)
  Gain24 : Gain  Gain=L5  Multiplication=Matrix(K*u)
  Gain25 : Gain  Gain=C2_cont  Multiplication=Matrix(K*u)
  Gain26 : Gain  Gain=-1
  Memory5 : Memory
  Square Root1 : Sqrt  SaturateOnIntegerOverflow=on
  Square2 : Math  Operator=square  SignedPower=off  SaturateOnIntegerOverflow=on
  Square3 : Math  Operator=square  SignedPower=off  SaturateOnIntegerOverflow=on
  Sum19 : Sum  Inputs=|+-
  Sum20 : Sum  Inputs=|++
  Sum21 : Sum  Inputs=|++
  Sum22 : Sum  Inputs=|+-
  Sum23 : Sum  Inputs=|++
  theta_wiener : Outport
  wires:
  Sum23/1 -> Square Root1/1
  Sum22/1 -> Gain24/1
  q/1 -> Gain21/1, Gain23/1  "u"
  Square3/1 -> Sum23/2
  Discrete-Time Integrator4/1 -> Gain22/1, Gain25/1, theta_wiener/1  "xe"
  Gain24/1 -> Sum21/2  "L(y-Cx-Du)"
  Square2/1 -> Sum23/1
  Square Root1/1 -> Divide4/2
  Divide4/1 -> Sum19/1  "theta"
  "wdotnobias = az "/1 -> Square3/1
  vdot = ay/1 -> Square2/1
  Memory5/1 -> Discrete-Time Integrator4/1
  udot = ax/1 -> Gain26/1
  Sum20/1 -> Sum21/1
  Gain25/1 -> Sum22/2  "Cx"
  Sum21/1 -> Memory5/1
  Gain26/1 -> Divide4/1
  Gain21/1 -> Sum19/2  "Du"
  Gain22/1 -> Sum20/1  "Axe"
  Sum19/1 -> Sum22/1
  Gain23/1 -> Sum20/2  "Bu"

== system HW7_v1/u wiener filter ==
  udot = ax : Inport
  u : Inport  Port=2
  Discrete-Time Integrator1 : DiscreteIntegrator  IntegratorMethod=Integration: Backward Euler  SampleTime=-1  ICPrevOutput=DiscIntNeverNeededParam  ICPrevScaledInput=DiscIntNeverNeededParam
  Gain10 : Gain  Gain=D2_cont  Multiplication=Matrix(K*u)
  Gain5 : Gain  Gain=A2_cont  Multiplication=Matrix(K*u)
  Gain7 : Gain  Gain=B2_cont  Multiplication=Matrix(K*u)
  Gain8 : Gain  Gain=L2  Multiplication=Matrix(K*u)
  Gain9 : Gain  Gain=C2_cont  Multiplication=Matrix(K*u)
  Memory2 : Memory
  Sum10 : Sum  Inputs=|+-
  Sum6 : Sum  Inputs=|++
  Sum8 : Sum  Inputs=|++
  Sum9 : Sum  Inputs=|+-
  "uwiener " : Outport
  wires:
  Gain7/1 -> Sum6/2  "Bu"
  Discrete-Time Integrator1/1 -> Gain5/1, Gain9/1, "uwiener "/1  "xe"
  Memory2/1 -> Discrete-Time Integrator1/1
  u/1 -> Sum10/1
  Gain9/1 -> Sum9/2  "Cx"
  Sum6/1 -> Sum8/1
  Sum8/1 -> Memory2/1
  Gain8/1 -> Sum8/2  "L(y-Cx-Du)"
  Sum10/1 -> Sum9/1
  Sum9/1 -> Gain8/1
  udot = ax/1 -> Gain10/1, Gain7/1  "u"
  Gain5/1 -> Sum6/1  "Axe"
  Gain10/1 -> Sum10/2  "Du"

== system HW7_v1/v wiener filter ==
  vdot = ay : Inport
  v : Inport  Port=2
  Discrete-Time Integrator2 : DiscreteIntegrator  IntegratorMethod=Integration: Backward Euler  SampleTime=-1  ICPrevOutput=DiscIntNeverNeededParam  ICPrevScaledInput=DiscIntNeverNeededParam
  Gain11 : Gain  Gain=D2_cont  Multiplication=Matrix(K*u)
  Gain12 : Gain  Gain=A2_cont  Multiplication=Matrix(K*u)
  Gain13 : Gain  Gain=B2_cont  Multiplication=Matrix(K*u)
  Gain14 : Gain  Gain=L3  Multiplication=Matrix(K*u)
  Gain15 : Gain  Gain=C2_cont  Multiplication=Matrix(K*u)
  Memory3 : Memory
  Sum11 : Sum  Inputs=|+-
  Sum12 : Sum  Inputs=|++
  Sum13 : Sum  Inputs=|++
  Sum14 : Sum  Inputs=|+-
  vwiener : Outport
  wires:
  v/1 -> Sum11/1
  vdot = ay/1 -> Gain11/1, Gain13/1  "u"
  Sum14/1 -> Gain14/1
  Gain11/1 -> Sum11/2  "Du"
  Gain14/1 -> Sum13/2  "L(y-Cx-Du)"
  Discrete-Time Integrator2/1 -> Gain12/1, Gain15/1, vwiener/1  "xe"
  Sum11/1 -> Sum14/1
  Memory3/1 -> Discrete-Time Integrator2/1
  Sum13/1 -> Memory3/1
  Gain13/1 -> Sum12/2  "Bu"
  Gain12/1 -> Sum12/1  "Axe"
  Sum12/1 -> Sum13/1
  Gain15/1 -> Sum14/2  "Cx"

== system HW7_v1/zw wiener filter ==
  note: zw Wiener Filter
  az : Inport
  z : Inport  Port=2
  Discrete-Time Integrator : DiscreteIntegrator  SampleTime=-1  ICPrevOutput=DiscIntNeverNeededParam  ICPrevScaledInput=DiscIntNeverNeededParam
  Gain1 : Gain  Gain=A1_wiener  Multiplication=Matrix(K*u)
  Gain2 : Gain  Gain=B1_wiener  Multiplication=Matrix(K*u)
  Gain3 : Gain  Gain=L1  Multiplication=Matrix(K*u)
  Gain4 : Gain  Gain=C1_wiener  Multiplication=Matrix(K*u)
  Gain6 : Gain  Gain=D1_wiener  Multiplication=Matrix(K*u)
  Sum3 : Sum  Inputs=+++
  Sum7 : Sum  Inputs=-+-
  zw_wiener : Outport
  wires:
  Gain3/1 -> Sum3/3  "L(y-Cx-Du)"
  Gain1/1 -> Sum3/1  "Axe"
  Gain2/1 -> Sum3/2  "Bu"
  Discrete-Time Integrator/1 -> zw_wiener/1, Gain1/1, Gain4/1  "xe"
  Gain6/1 -> Sum7/1  "Du"
  az/1 -> Gain6/1, Gain2/1  "u = az"
  Sum7/1 -> Gain3/1
  z/1 -> Sum7/2  "Zned"
  Gain4/1 -> Sum7/3  "Cx"
  Sum3/1 -> Discrete-Time Integrator/1

== system HW7_v1/zw wiener filter2 ==
  note: zw Wiener Filter
  az : Inport
  z : Inport  Port=2
  Discrete-Time Integrator : DiscreteIntegrator  SampleTime=-1  ICPrevOutput=DiscIntNeverNeededParam  ICPrevScaledInput=DiscIntNeverNeededParam
  Gain1 : Gain  Gain=A1_wiener  Multiplication=Matrix(K*u)
  Gain2 : Gain  Gain=B1_wiener  Multiplication=Matrix(K*u)
  Gain3 : Gain  Gain=L1  Multiplication=Matrix(K*u)
  Gain4 : Gain  Gain=C1_wiener  Multiplication=Matrix(K*u)
  Gain6 : Gain  Gain=D1_wiener  Multiplication=Matrix(K*u)
  Sum3 : Sum  Inputs=+++
  Sum7 : Sum  Inputs=-+-
  zw_wiener : Outport
  wires:
  Gain3/1 -> Sum3/3  "L(y-Cx-Du)"
  Gain1/1 -> Sum3/1  "Axe"
  Gain2/1 -> Sum3/2  "Bu"
  Discrete-Time Integrator/1 -> zw_wiener/1, Gain1/1, Gain4/1  "xe"
  Gain6/1 -> Sum7/1  "Du"
  az/1 -> Gain6/1, Gain2/1  "u = az"
  Sum7/1 -> Gain3/1
  z/1 -> Sum7/2  "Zned"
  Gain4/1 -> Sum7/3  "Cx"
  Sum3/1 -> Discrete-Time Integrator/1

== system HW7_v1/Nonlinear System/Acceleration ==
  n1 : Inport
  n2 : Inport  Port=2
  n3 : Inport  Port=3
  n4 : Inport  Port=4
  Gain : Gain  Gain=1.9060e-06
  Square{,1..3} (4 alike) : Math  Operator=square  SignedPower=off  SaturateOnIntegerOverflow=on
  Sum : Sum  Inputs=----
  az : Outport
  wires:
  n1/1 -> Square/1
  n2/1 -> Square1/1
  n3/1 -> Square2/1
  n4/1 -> Square3/1
  Square/1 -> Sum/1
  Square1/1 -> Sum/2
  Square2/1 -> Sum/3
  Square3/1 -> Sum/4
  Sum/1 -> Gain/1
  Gain/1 -> az/1

== system HW7_v1/Nonlinear System/Height ==
  "ZNED_in " : Inport
  Gain : Gain  Gain=-1
  "h_out " : Outport
  wires:
  "ZNED_in "/1 -> Gain/1
  Gain/1 -> "h_out "/1

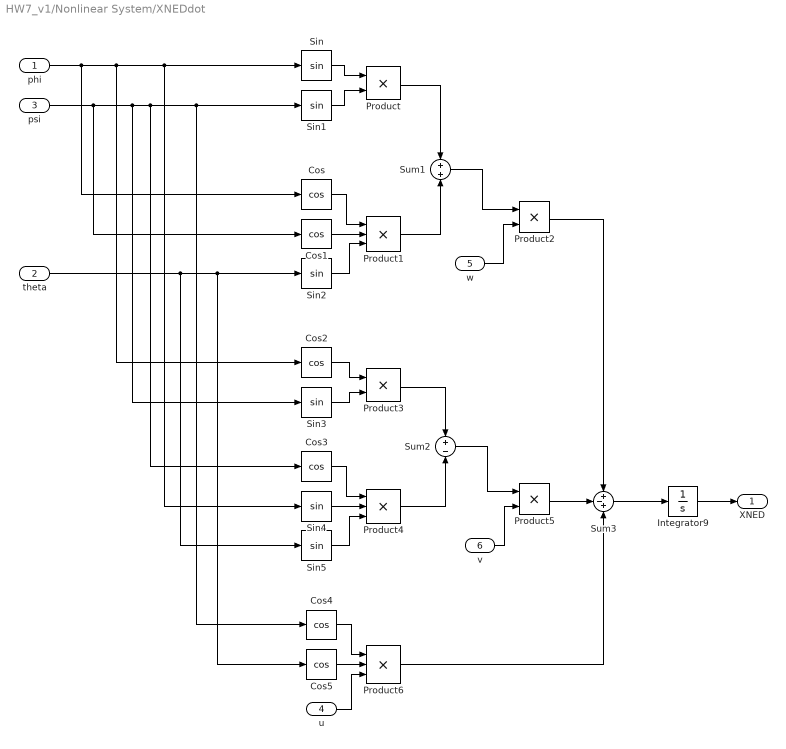
== system HW7_v1/Nonlinear System/XNEDdot  ==
  phi : Inport
  theta : Inport  Port=2
  psi : Inport  Port=3
  u : Inport  Port=4
  w : Inport  Port=5
  v : Inport  Port=6
  Cos{,1..5} (6 alike) : Trigonometry  Operator=cos
  Integrator9 : Integrator
  Product{,2..3,5} (4 alike) : Product
  Product1 : Product  Inputs=3
  Product4 : Product  Inputs=3
  Product6 : Product  Inputs=3
  Sin{,1..5} (6 alike) : Trigonometry
  Sum1 : Sum
  Sum2 : Sum  Inputs=+-
  Sum3 : Sum  Inputs=+-+
  XNED : Outport
  wires:
  Cos1/1 -> Product1/2
  Sum1/1 -> Product2/1
  Product1/1 -> Sum1/2
  Product/1 -> Sum1/1
  Sin1/1 -> Product/2
  Sin/1 -> Product/1
  Cos/1 -> Product1/1
  Sin2/1 -> Product1/3
  w/1 -> Product2/2
  Product4/1 -> Sum2/2
  v/1 -> Product5/2
  Product3/1 -> Sum2/1
  Sum2/1 -> Product5/1
  Cos5/1 -> Product6/2
  u/1 -> Product6/3
  Product2/1 -> Sum3/1
  Product5/1 -> Sum3/2
  Product6/1 -> Sum3/3
  Sum3/1 -> Integrator9/1
  Integrator9/1 -> XNED/1
  Cos2/1 -> Product3/1
  Sin3/1 -> Product3/2
  Cos3/1 -> Product4/1
  phi/1 -> Cos2/1, Sin4/1, Sin/1, Cos/1
  Sin4/1 -> Product4/2
  Sin5/1 -> Product4/3
  psi/1 -> Cos1/1, Sin3/1, Cos3/1, Cos4/1, Sin1/1
  Cos4/1 -> Product6/1
  theta/1 -> Sin5/1, Cos5/1, Sin2/1

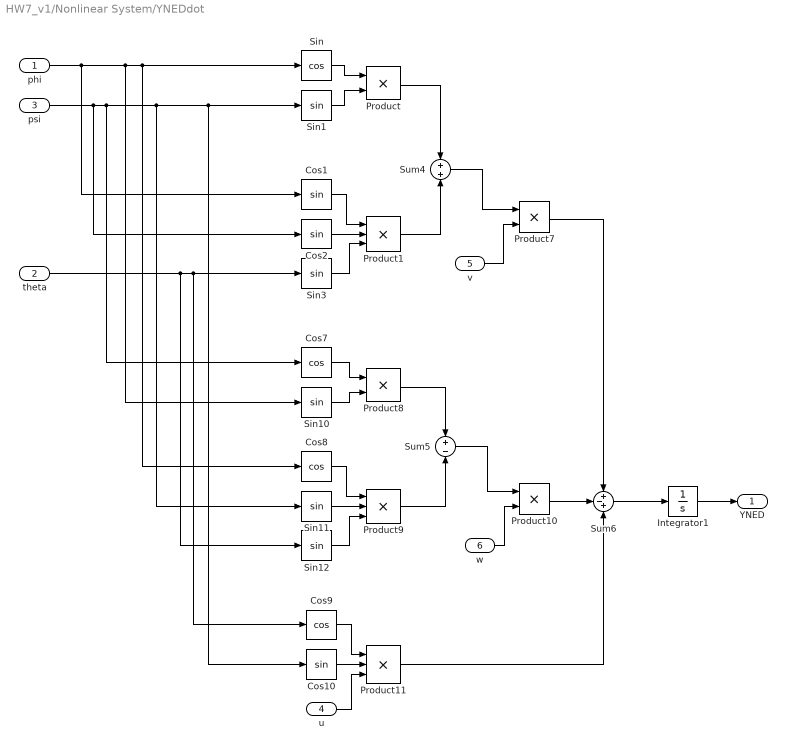
== system HW7_v1/Nonlinear System/YNEDdot  ==
  phi : Inport
  theta : Inport  Port=2
  psi : Inport  Port=3
  u : Inport  Port=4
  v : Inport  Port=5
  w : Inport  Port=6
  Cos1 : Trigonometry
  Cos10 : Trigonometry
  Cos2 : Trigonometry
  Cos7 : Trigonometry  Operator=cos
  Cos8 : Trigonometry  Operator=cos
  Cos9 : Trigonometry  Operator=cos
  Integrator1 : Integrator
  Product{,7..8,10} (4 alike) : Product
  Product1 : Product  Inputs=3
  Product11 : Product  Inputs=3
  Product9 : Product  Inputs=3
  Sin : Trigonometry  Operator=cos
  Sin{1,3,10..12} (5 alike) : Trigonometry
  Sum4 : Sum
  Sum5 : Sum  Inputs=+-
  Sum6 : Sum  Inputs=+-+
  YNED : Outport
  wires:
  Sin/1 -> Product/1
  Cos7/1 -> Product8/1
  Sin11/1 -> Product9/2
  Sin12/1 -> Product9/3
  Product9/1 -> Sum5/2
  Sin10/1 -> Product8/2
  Sum5/1 -> Product10/1
  Product11/1 -> Sum6/3
  Sum6/1 -> Integrator1/1
  Product8/1 -> Sum5/1
  Product10/1 -> Sum6/2
  Product7/1 -> Sum6/1
  Sin3/1 -> Product1/3
  Cos1/1 -> Product1/1
  Product/1 -> Sum4/1
  Product1/1 -> Sum4/2
  Cos2/1 -> Product1/2
  v/1 -> Product7/2
  Cos9/1 -> Product11/1
  theta/1 -> Sin12/1, Cos9/1, Sin3/1
  Sin1/1 -> Product/2
  Sum4/1 -> Product7/1
  u/1 -> Product11/3
  w/1 -> Product10/2
  phi/1 -> Sin10/1, Cos8/1, Sin/1, Cos1/1
  psi/1 -> Cos2/1, Cos7/1, Sin11/1, Cos10/1, Sin1/1
  Cos8/1 -> Product9/1
  Integrator1/1 -> YNED/1
  Cos10/1 -> Product11/2

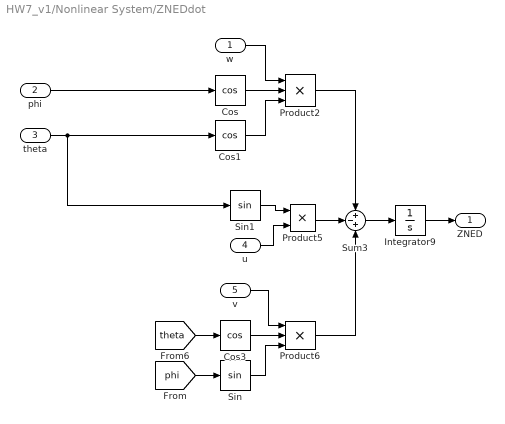
== system HW7_v1/Nonlinear System/ZNEDdot ==
  w : Inport
  phi : Inport  Port=2
  theta : Inport  Port=3
  u : Inport  Port=4
  v : Inport  Port=5
  Cos : Trigonometry  Operator=cos
  Cos1 : Trigonometry  Operator=cos
  Cos3 : Trigonometry  Operator=cos
  Integrator9 : Integrator
  Product2 : Product  Inputs=3
  Product5 : Product
  Product6 : Product  Inputs=3
  Sin : Trigonometry
  Sin1 : Trigonometry
  Sum3 : Sum  Inputs=+-+
  ZNED : Outport
  wires:
  Product6/1 -> Sum3/3
  [phi] -> Sin/1
  Sum3/1 -> Integrator9/1
  Product2/1 -> Sum3/1
  Product5/1 -> Sum3/2
  u/1 -> Product5/2
  Integrator9/1 -> ZNED/1
  theta/1 -> Cos1/1, Sin1/1
  Cos/1 -> Product2/2
  Cos1/1 -> Product2/3
  Sin1/1 -> Product5/1
  phi/1 -> Cos/1
  [theta] -> Cos3/1
  w/1 -> Product2/1
  Cos3/1 -> Product6/2
  Sin/1 -> Product6/3
  v/1 -> Product6/1

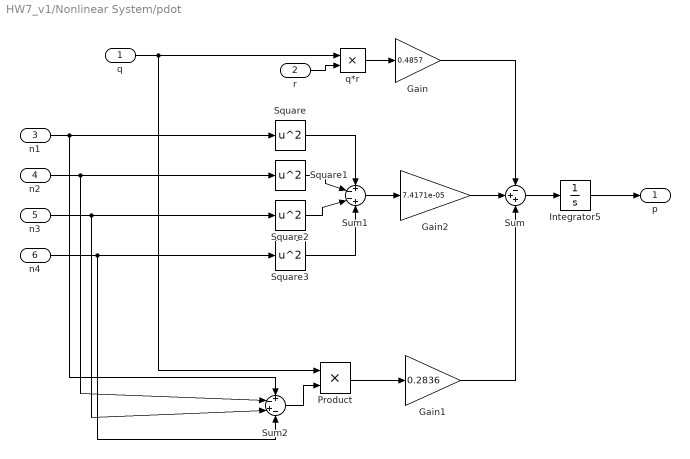
== system HW7_v1/Nonlinear System/pdot ==
  q : Inport
  r : Inport  Port=2
  n1 : Inport  Port=3
  n2 : Inport  Port=4
  n3 : Inport  Port=5
  n4 : Inport  Port=6
  Gain : Gain  Gain=0.4857
  Gain1 : Gain  Gain=0.2836
  Gain2 : Gain  Gain=7.4171e-05
  Integrator5 : Integrator
  Product : Product
  Square{,1..3} (4 alike) : Math  Operator=square  SignedPower=off  SaturateOnIntegerOverflow=on
  Sum : Sum  Inputs=-++
  Sum1 : Sum  Inputs=+--+
  Sum2 : Sum  Inputs=+-+-
  q*r : Product
  p : Outport
  wires:
  Square1/1 -> Sum1/2
  Sum/1 -> Integrator5/1
  Square2/1 -> Sum1/3
  Square/1 -> Sum1/1
  Integrator5/1 -> p/1
  Square3/1 -> Sum1/4
  r/1 -> q*r/2
  q*r/1 -> Gain/1
  Sum1/1 -> Gain2/1
  Sum2/1 -> Product/2
  Product/1 -> Gain1/1
  Gain1/1 -> Sum/3
  n1/1 -> Sum2/1, Square/1
  n4/1 -> Square3/1, Sum2/4
  n3/1 -> Square2/1, Sum2/3
  n2/1 -> Sum2/2, Square1/1
  q/1 -> Product/1, q*r/1
  Gain/1 -> Sum/1
  Gain2/1 -> Sum/2

== system HW7_v1/Nonlinear System/phidot ==
  p : Inport
  r : Inport  Port=2
  theta : Inport  Port=3
  q : Inport  Port=4
  phi in : Inport  Port=5
  Cos : Trigonometry  Operator=cos
  Cos1 : Trigonometry  Operator=cos
  Integrator9 : Integrator
  Product : Product
  Product1 : Product
  Product2 : Product
  Sum : Sum
  Sum1 : Sum
  Tan : Trigonometry  Operator=tan
  phi : Outport
  wires:
  Integrator9/1 -> phi/1  "phi"
  theta/1 -> Tan/1
  p/1 -> Sum/1
  q/1 -> Product1/1
  r/1 -> Product/1
  Cos/1 -> Product/2
  Product/1 -> Sum1/1
  Product1/1 -> Sum1/2
  Tan/1 -> Product2/1
  Sum1/1 -> Product2/2
  Product2/1 -> Sum/2
  Sum/1 -> Integrator9/1
  Cos1/1 -> Product1/2
  phi in/1 -> Cos1/1, Cos/1

== system HW7_v1/Nonlinear System/psidot  ==
  r : Inport
  phi : Inport  Port=2
  q : Inport  Port=3
  theta : Inport  Port=4
  1/cos(theta) : Fcn  Expr=1/cos(u)
  Cos : Trigonometry  Operator=cos
  Integrator9 : Integrator
  Product : Product
  Product1 : Product
  Product2 : Product
  Sin : Trigonometry
  Sum1 : Sum
  psi : Outport
  wires:
  q/1 -> Product1/1
  Cos/1 -> Product/2
  Product1/1 -> Sum1/2
  Integrator9/1 -> psi/1
  Sin/1 -> Product1/2
  Product/1 -> Sum1/1
  r/1 -> Product/1
  Sum1/1 -> Product2/1
  theta/1 -> 1/cos(theta)/1
  1/cos(theta)/1 -> Product2/2
  Product2/1 -> Integrator9/1
  phi/1 -> Sin/1, Cos/1

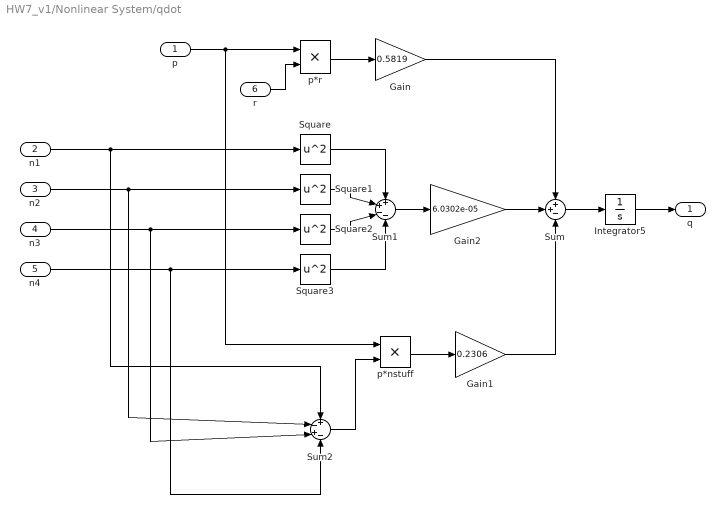
== system HW7_v1/Nonlinear System/qdot ==
  p : Inport
  n1 : Inport  Port=2
  n2 : Inport  Port=3
  n3 : Inport  Port=4
  n4 : Inport  Port=5
  r : Inport  Port=6
  Gain : Gain  Gain=0.5819
  Gain1 : Gain  Gain=0.2306
  Gain2 : Gain  Gain=6.0302e-05
  Integrator5 : Integrator
  Square{,1..3} (4 alike) : Math  Operator=square  SignedPower=off  SaturateOnIntegerOverflow=on
  Sum : Sum  Inputs=++-
  Sum1 : Sum  Inputs=++--
  Sum2 : Sum  Inputs=+-+-
  p*nstuff : Product
  p*r : Product
  q : Outport
  wires:
  Sum/1 -> Integrator5/1
  Gain1/1 -> Sum/3
  n2/1 -> Sum2/2, Square1/1
  r/1 -> p*r/2
  Square3/1 -> Sum1/4
  Square1/1 -> Sum1/2
  p*nstuff/1 -> Gain1/1
  Integrator5/1 -> q/1
  p*r/1 -> Gain/1
  Square/1 -> Sum1/1
  Sum1/1 -> Gain2/1
  Square2/1 -> Sum1/3
  Sum2/1 -> p*nstuff/2
  Gain2/1 -> Sum/2
  Gain/1 -> Sum/1
  n4/1 -> Square3/1, Sum2/4
  n1/1 -> Sum2/1, Square/1
  n3/1 -> Square2/1, Sum2/3
  p/1 -> p*nstuff/1, p*r/1

== system HW7_v1/Nonlinear System/rdot ==
  p : Inport
  n1 : Inport  Port=2
  n2 : Inport  Port=3
  n3 : Inport  Port=4
  n4 : Inport  Port=5
  q : Inport  Port=6
  Gain : Gain  Gain=0.1341
  Gain2 : Gain  Gain=7.2236e-05
  Integrator5 : Integrator
  Square{,1..3} (4 alike) : Math  Operator=square  SignedPower=off  SaturateOnIntegerOverflow=on
  Sum : Sum  Inputs=-+
  Sum1 : Sum  Inputs=-+-+
  p*q : Product
  r : Outport
  wires:
  n3/1 -> Square2/1
  Gain/1 -> Sum/1
  n4/1 -> Square3/1
  q/1 -> p*q/2
  Square/1 -> Sum1/1
  p*q/1 -> Gain/1
  Square1/1 -> Sum1/2
  Sum/1 -> Integrator5/1
  p/1 -> p*q/1
  n2/1 -> Square1/1
  n1/1 -> Square/1
  Sum1/1 -> Gain2/1
  Square2/1 -> Sum1/3
  Square3/1 -> Sum1/4
  Gain2/1 -> Sum/2
  Integrator5/1 -> r/1

== system HW7_v1/Nonlinear System/thetadot  ==
  r : Inport
  phi : Inport  Port=2
  q : Inport  Port=3
  Cos : Trigonometry  Operator=cos
  Integrator9 : Integrator
  Product : Product
  Product1 : Product
  Sin : Trigonometry
  Sum1 : Sum  Inputs=+-
  theta : Outport
  wires:
  Cos/1 -> Product/2
  r/1 -> Product1/1
  Product1/1 -> Sum1/2
  Integrator9/1 -> theta/1  "theta"
  Sin/1 -> Product1/2
  Product/1 -> Sum1/1
  q/1 -> Product/1
  Sum1/1 -> Integrator9/1
  phi/1 -> Sin/1, Cos/1

== system HW7_v1/Nonlinear System/udot ==
  "q " : Inport
  "w " : Inport  Port=2
  theta : Inport  Port=3
  "r " : Inport  Port=4
  v : Inport  Port=5
  Gain : Gain  Gain=9.81
  Integrator5 : Integrator
  Sin : Trigonometry
  Sum : Sum  Inputs=+--
  q*w : Product
  r*v : Product
  "u " : Outport
  wires:
  Integrator5/1 -> "u "/1  "u"
  "q "/1 -> q*w/1
  "w "/1 -> q*w/2
  q*w/1 -> Sum/1
  theta/1 -> Sin/1
  Sin/1 -> Gain/1
  Gain/1 -> Sum/2
  "r "/1 -> r*v/1
  v/1 -> r*v/2
  r*v/1 -> Sum/3
  Sum/1 -> Integrator5/1

== system HW7_v1/Nonlinear System/vdot ==
  theta : Inport
  phi : Inport  Port=2
  p : Inport  Port=3
  w : Inport  Port=4
  r : Inport  Port=5
  u : Inport  Port=6
  Constant : Constant  Value=9.81  SampleTime=0.05
  Cos : Trigonometry  Operator=cos
  Integrator5 : Integrator
  Product : Product  Inputs=3
  Sin : Trigonometry
  Sum : Sum  Inputs=+-+
  p*w : Product
  r*u : Product
  v : Outport
  wires:
  r/1 -> r*u/1
  p/1 -> p*w/1
  Sum/1 -> Integrator5/1
  Integrator5/1 -> v/1  "v"
  w/1 -> p*w/2
  u/1 -> r*u/2
  r*u/1 -> Sum/3
  theta/1 -> Cos/1
  Cos/1 -> Product/2
  Sin/1 -> Product/3
  phi/1 -> Sin/1
  Product/1 -> Sum/1
  p*w/1 -> Sum/2
  Constant/1 -> Product/1

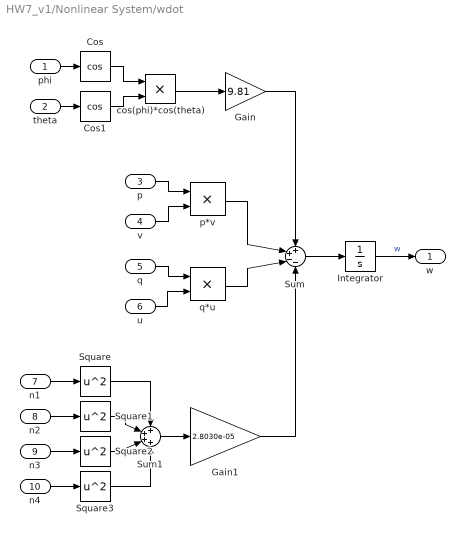
== system HW7_v1/Nonlinear System/wdot  ==
  phi : Inport
  theta : Inport  Port=2
  p : Inport  Port=3
  v : Inport  Port=4
  q : Inport  Port=5
  u : Inport  Port=6
  n1 : Inport  Port=7
  n2 : Inport  Port=8
  n3 : Inport  Port=9
  n4 : Inport  Port=10
  Cos : Trigonometry  Operator=cos
  Cos1 : Trigonometry  Operator=cos
  Gain : Gain  Gain=9.81
  Gain1 : Gain  Gain=2.8030e-05
  Integrator : Integrator
  Square{,1..3} (4 alike) : Math  Operator=square  SignedPower=off  SaturateOnIntegerOverflow=on
  Sum : Sum  Inputs=++--
  Sum1 : Sum  Inputs=++++
  cos(phi)*cos(theta) : Product
  p*v : Product
  q*u : Product
  w : Outport
  wires:
  q*u/1 -> Sum/3
  u/1 -> q*u/2
  Integrator/1 -> w/1  "w"
  Gain/1 -> Sum/1
  q/1 -> q*u/1
  Sum/1 -> Integrator/1
  v/1 -> p*v/2
  p/1 -> p*v/1
  p*v/1 -> Sum/2
  theta/1 -> Cos1/1
  Cos1/1 -> cos(phi)*cos(theta)/2
  Cos/1 -> cos(phi)*cos(theta)/1
  cos(phi)*cos(theta)/1 -> Gain/1
  phi/1 -> Cos/1
  n1/1 -> Square/1
  Gain1/1 -> Sum/4
  Square/1 -> Sum1/1
  n2/1 -> Square1/1
  n3/1 -> Square2/1
  n4/1 -> Square3/1
  Square1/1 -> Sum1/2
  Square2/1 -> Sum1/3
  Square3/1 -> Sum1/4
  Sum1/1 -> Gain1/1
